simulink library "_system"
libraries: AtomicLibrary x5, BusImpl x1

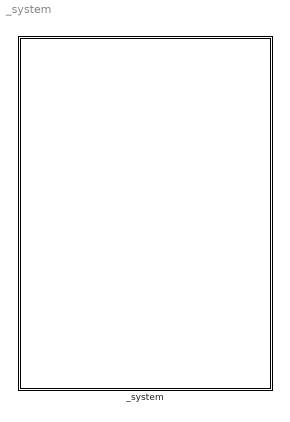
== system _system ==
  _system : Subsystem  Tag=id=_75GNMfUnEeOqvInL61-gjw

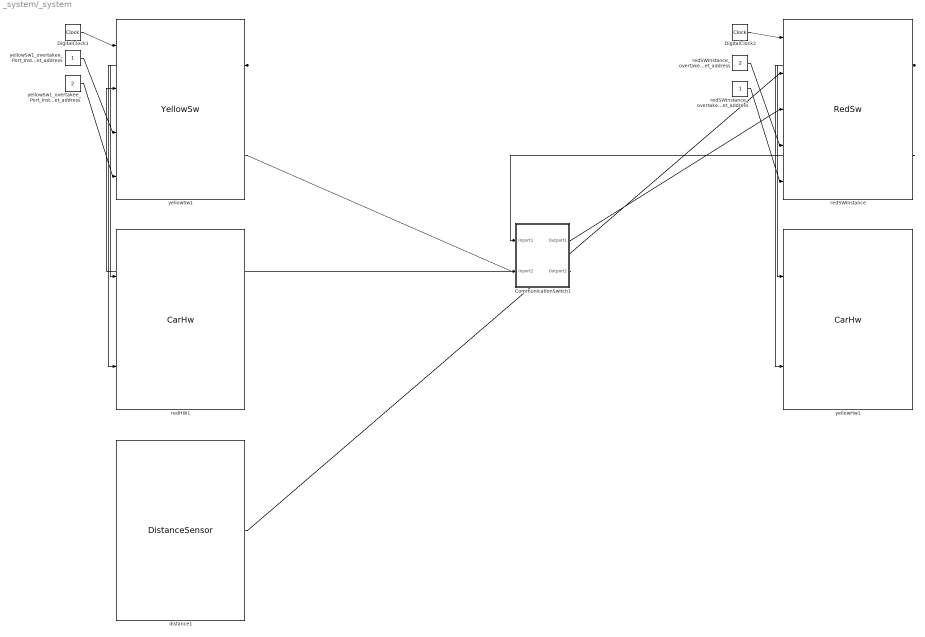
== system _system/_system ==
  CommunicationSwitch1 : Subsystem  Tag=id=_75PXIPUnEeOqvInL61-gjw  LoadFcn=MainBusGenerator
  yellowSw1 : AtomicLibrary/YellowSw  Tag=id=_75iSEPUnEeOqvInL61-gjw
  DigitalClock1 : DigitalClock  Tag=id=_75iSEfUnEeOqvInL61-gjw  SampleTime=0.001
  redSWInstance : AtomicLibrary/RedSw  Tag=id=_75sDEPUnEeOqvInL61-gjw
  DigitalClock2 : DigitalClock  Tag=id=_75sDEfUnEeOqvInL61-gjw  SampleTime=0.001
  redHW1 : AtomicLibrary/CarHw  Tag=id=_75--APUnEeOqvInL61-gjw
  yellowHw1 : AtomicLibrary/CarHw  Tag=id=_75--AfUnEeOqvInL61-gjw
  distance1 : AtomicLibrary/DistanceSensor  Tag=id=_76IvAPUnEeOqvInL61-gjw
  yellowSw1_overtakee_Port_Instance_net_address : Constant  Tag=id=_8DqecPUnEeOqvInL61-gjw  Value=1  OutDataTypeMode=uint8  OutDataTypeStr=uint8
  redSWInstance_overtaker_Port_Instance_net_address : Constant  Tag=id=_8D0PcPUnEeOqvInL61-gjw  Value=2  OutDataTypeMode=uint8  OutDataTypeStr=uint8
  redSWInstance_overtaker_Port_Instance_receiver_net_address : Constant  Tag=id=_8FmYJfUnEeOqvInL61-gjw  Value=1  OutDataTypeMode=uint8  OutDataTypeStr=uint8
  yellowSw1_overtakee_Port_Instance_receiver_net_address : Constant  Tag=id=_8FwJIfUnEeOqvInL61-gjw  Value=2  OutDataTypeMode=uint8  OutDataTypeStr=uint8
  wires:
  DigitalClock1/1 -> yellowSw1/1
  DigitalClock2/1 -> redSWInstance/1
  yellowSw1_overtakee_Port_Instance_net_address/1 -> yellowSw1/3
  redSWInstance_overtaker_Port_Instance_net_address/1 -> redSWInstance/4
  yellowSw1/1 -> redHW1/1, redHW1/2
  redSWInstance/1 -> yellowHw1/1, yellowHw1/2
  distance1/1 -> redSWInstance/2
  redSWInstance/2 -> CommunicationSwitch1/1(Inport1)
  yellowSw1/2 -> CommunicationSwitch1/2(Inport2)
  CommunicationSwitch1/2(Outport2) -> yellowSw1/2
  CommunicationSwitch1/1(Outport1) -> redSWInstance/3
  redSWInstance_overtaker_Port_Instance_receiver_net_address/1 -> redSWInstance/5
  yellowSw1_overtakee_Port_Instance_receiver_net_address/1 -> yellowSw1/4

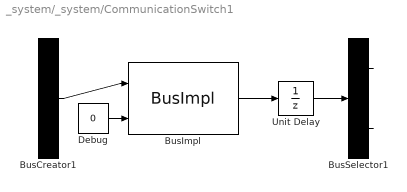
== system _system/_system/CommunicationSwitch1 ==
  Inport1 : Inport  Tag=id=_8FwJIvUnEeOqvInL61-gjw  Port=1  DataType=auto  OutDataType=fixdt(1, 16)  OutScaling=2^0  UseBusObject=on  OutDataTypeStr=Inherit: auto
      settings: BusObject=PacketBus
  Inport2 : Inport  Tag=id=_8FwJJPUnEeOqvInL61-gjw  Port=2  DataType=auto  OutDataType=fixdt(1, 16)  OutScaling=2^0  UseBusObject=on  OutDataTypeStr=Inherit: auto
      settings: BusObject=PacketBus
  Outport1 : Outport  Tag=id=_8FwJI_UnEeOqvInL61-gjw  Port=1  DataType=auto  OutDataType=fixdt(1, 16)  OutScaling=2^0  UseBusObject=on  OutDataTypeStr=Inherit: auto
      settings: BusObject=PacketBus
  Outport2 : Outport  Tag=id=_8FwJJfUnEeOqvInL61-gjw  Port=2  DataType=auto  OutDataType=fixdt(1, 16)  OutScaling=2^0  UseBusObject=on  OutDataTypeStr=Inherit: auto
      settings: BusObject=PacketBus
  BusCreator1 : BusCreator  Inputs=2  UseBusObject=on
      settings: BusObject=MainBus
  BusSelector1 : BusSelector  OutputSignals=rc1,rc2
  Unit Delay : UnitDelay  SampleTime=-1
  BusImpl : BusImpl/BusImpl
  Debug : Constant  Value=0  OutDataType=fixdt(1, 16)  OutScaling=2^0
  wires:
  BusImpl/1 -> Unit Delay/1
  BusCreator1/1 -> BusImpl/1
  Unit Delay/1 -> BusSelector1/1
  Inport1/1 -> BusCreator1/1  "rc1"
  Inport2/1 -> BusCreator1/2  "rc2"
  BusSelector1/1 -> Outport1/1
  BusSelector1/2 -> Outport2/1
  Debug/1 -> BusImpl/2
